simulink model "cuurent_controlled_circuit"  (R2022a)
settings: Solver=VariableStepAuto  StartTime=0.0  StopTime=25.0  RelTol=1e-3
undefined symbols (not defined in the file or in its folder): DiscIntNeverNeededParam
libraries: fl_lib x82, nesl_utility x65, eeRmsMeasurement x34, eePowerMeasurement x17, ee_lib x16
(part 3 of 3)

== system cuurent_controlled_circuit/Subsystem5 ==
  Display3 : Display
  Display4 : Display
  Display5 : Display
  PS-Simulink Converter2 : nesl_utility/PS-Simulink Converter  PhysicalDomain=network_engine_domain  SubClassName=ps_output  LeftPortType=input  RightPortType=output  PseudoPeriodic=off  Frequencies=[]  VectorFormat=inherit  Unit=inherit  AffineConversion=off
      settings: SourceProductBaseCode=SS,PW,VE
  PS-Simulink Converter3 : nesl_utility/PS-Simulink Converter  PhysicalDomain=network_engine_domain  SubClassName=ps_output  LeftPortType=input  RightPortType=output  PseudoPeriodic=off  Frequencies=[]  VectorFormat=inherit  Unit=inherit  AffineConversion=off
      settings: SourceProductBaseCode=SS,PW,VE
  Power Measurement2 : eePowerMeasurement/Power Measurement  LabelModeActiveChoice=Continuous  F=50  K=[0 1 2 3]  Ts=0
      settings: SourceProductBaseCode=PS
  RMS Measurement2 : eeRmsMeasurement/RMS Measurement  LabelModeActiveChoice=Total  F=50  SpecifyHarmonics=off  K=[0 1 2]  Ts=0
      settings: SourceProductBaseCode=PS
  RMS Measurement3 : eeRmsMeasurement/RMS Measurement  LabelModeActiveChoice=Total  F=50  SpecifyHarmonics=off  K=[0 1 2]  Ts=0
      settings: SourceProductBaseCode=PS
  Scope{6..10} (5 alike) : Scope
  input : PMIOPort  Side=Left
  input1 : PMIOPort  Port=2  Side=Left
  Q : Outport
  wires:
  Power Measurement2/2 -> Q/1
  PS-Simulink Converter3/1 -> RMS Measurement3/1, Scope8/1
  Power Measurement2/1 -> Display5/1, Scope10/1
  RMS Measurement2/1 -> Scope7/1, Display3/1, Power Measurement2/1
  PS-Simulink Converter2/1 -> RMS Measurement2/1, Scope6/1
  RMS Measurement3/1 -> Power Measurement2/2, Scope9/1, Display4/1
  connections:
  PS-Simulink Converter3/LConn1 -- input1/RConn1
  PS-Simulink Converter2/LConn1 -- input/RConn1

== system cuurent_controlled_circuit/Subsystem6 ==
  Display3 : Display
  Display4 : Display
  Display5 : Display
  PS-Simulink Converter2 : nesl_utility/PS-Simulink Converter  PhysicalDomain=network_engine_domain  SubClassName=ps_output  LeftPortType=input  RightPortType=output  PseudoPeriodic=off  Frequencies=[]  VectorFormat=inherit  Unit=inherit  AffineConversion=off
      settings: SourceProductBaseCode=SS,PW,VE
  PS-Simulink Converter3 : nesl_utility/PS-Simulink Converter  PhysicalDomain=network_engine_domain  SubClassName=ps_output  LeftPortType=input  RightPortType=output  PseudoPeriodic=off  Frequencies=[]  VectorFormat=inherit  Unit=inherit  AffineConversion=off
      settings: SourceProductBaseCode=SS,PW,VE
  Power Measurement2 : eePowerMeasurement/Power Measurement  LabelModeActiveChoice=Continuous  F=50  K=[0 1 2 3]  Ts=0
      settings: SourceProductBaseCode=PS
  RMS Measurement2 : eeRmsMeasurement/RMS Measurement  LabelModeActiveChoice=Total  F=50  SpecifyHarmonics=off  K=[0 1 2]  Ts=0
      settings: SourceProductBaseCode=PS
  RMS Measurement3 : eeRmsMeasurement/RMS Measurement  LabelModeActiveChoice=Total  F=50  SpecifyHarmonics=off  K=[0 1 2]  Ts=0
      settings: SourceProductBaseCode=PS
  Scope{6..10} (5 alike) : Scope
  input : PMIOPort  Side=Left
  input1 : PMIOPort  Port=2  Side=Left
  Q : Outport
  wires:
  Power Measurement2/2 -> Q/1
  PS-Simulink Converter3/1 -> RMS Measurement3/1, Scope8/1
  Power Measurement2/1 -> Display5/1, Scope10/1
  RMS Measurement2/1 -> Scope7/1, Display3/1, Power Measurement2/1
  PS-Simulink Converter2/1 -> RMS Measurement2/1, Scope6/1
  RMS Measurement3/1 -> Power Measurement2/2, Scope9/1, Display4/1
  connections:
  PS-Simulink Converter3/LConn1 -- input1/RConn1
  PS-Simulink Converter2/LConn1 -- input/RConn1

== system cuurent_controlled_circuit/Subsystem7 ==
  Display3 : Display
  Display4 : Display
  Display5 : Display
  PS-Simulink Converter2 : nesl_utility/PS-Simulink Converter  PhysicalDomain=network_engine_domain  SubClassName=ps_output  LeftPortType=input  RightPortType=output  PseudoPeriodic=off  Frequencies=[]  VectorFormat=inherit  Unit=inherit  AffineConversion=off
      settings: SourceProductBaseCode=SS,PW,VE
  PS-Simulink Converter3 : nesl_utility/PS-Simulink Converter  PhysicalDomain=network_engine_domain  SubClassName=ps_output  LeftPortType=input  RightPortType=output  PseudoPeriodic=off  Frequencies=[]  VectorFormat=inherit  Unit=inherit  AffineConversion=off
      settings: SourceProductBaseCode=SS,PW,VE
  Power Measurement2 : eePowerMeasurement/Power Measurement  LabelModeActiveChoice=Continuous  F=50  K=[0 1 2 3]  Ts=0
      settings: SourceProductBaseCode=PS
  RMS Measurement2 : eeRmsMeasurement/RMS Measurement  LabelModeActiveChoice=Total  F=50  SpecifyHarmonics=off  K=[0 1 2]  Ts=0
      settings: SourceProductBaseCode=PS
  RMS Measurement3 : eeRmsMeasurement/RMS Measurement  LabelModeActiveChoice=Total  F=50  SpecifyHarmonics=off  K=[0 1 2]  Ts=0
      settings: SourceProductBaseCode=PS
  Scope{6..10} (5 alike) : Scope
  input : PMIOPort  Side=Left
  input1 : PMIOPort  Port=2  Side=Left
  Q : Outport
  wires:
  Power Measurement2/2 -> Q/1
  PS-Simulink Converter3/1 -> RMS Measurement3/1, Scope8/1
  Power Measurement2/1 -> Display5/1, Scope10/1
  RMS Measurement2/1 -> Scope7/1, Display3/1, Power Measurement2/1
  PS-Simulink Converter2/1 -> RMS Measurement2/1, Scope6/1
  RMS Measurement3/1 -> Power Measurement2/2, Scope9/1, Display4/1
  connections:
  PS-Simulink Converter3/LConn1 -- input1/RConn1
  PS-Simulink Converter2/LConn1 -- input/RConn1

== system cuurent_controlled_circuit/Subsystem8 ==
  Display3 : Display
  Display4 : Display
  Display5 : Display
  PS-Simulink Converter2 : nesl_utility/PS-Simulink Converter  PhysicalDomain=network_engine_domain  SubClassName=ps_output  LeftPortType=input  RightPortType=output  PseudoPeriodic=off  Frequencies=[]  VectorFormat=inherit  Unit=inherit  AffineConversion=off
      settings: SourceProductBaseCode=SS,PW,VE
  PS-Simulink Converter3 : nesl_utility/PS-Simulink Converter  PhysicalDomain=network_engine_domain  SubClassName=ps_output  LeftPortType=input  RightPortType=output  PseudoPeriodic=off  Frequencies=[]  VectorFormat=inherit  Unit=inherit  AffineConversion=off
      settings: SourceProductBaseCode=SS,PW,VE
  Power Measurement2 : eePowerMeasurement/Power Measurement  LabelModeActiveChoice=Continuous  F=50  K=[0 1 2 3]  Ts=0
      settings: SourceProductBaseCode=PS
  RMS Measurement2 : eeRmsMeasurement/RMS Measurement  LabelModeActiveChoice=Total  F=50  SpecifyHarmonics=off  K=[0 1 2]  Ts=0
      settings: SourceProductBaseCode=PS
  RMS Measurement3 : eeRmsMeasurement/RMS Measurement  LabelModeActiveChoice=Total  F=50  SpecifyHarmonics=off  K=[0 1 2]  Ts=0
      settings: SourceProductBaseCode=PS
  Scope{6..10} (5 alike) : Scope
  input : PMIOPort  Side=Left
  input1 : PMIOPort  Port=2  Side=Left
  Q : Outport
  wires:
  Power Measurement2/2 -> Q/1
  PS-Simulink Converter3/1 -> RMS Measurement3/1, Scope8/1
  Power Measurement2/1 -> Display5/1, Scope10/1
  RMS Measurement2/1 -> Scope7/1, Display3/1, Power Measurement2/1
  PS-Simulink Converter2/1 -> RMS Measurement2/1, Scope6/1
  RMS Measurement3/1 -> Power Measurement2/2, Scope9/1, Display4/1
  connections:
  PS-Simulink Converter3/LConn1 -- input1/RConn1
  PS-Simulink Converter2/LConn1 -- input/RConn1

== system cuurent_controlled_circuit/Subsystem9 ==
  Display3 : Display
  Display4 : Display
  Display5 : Display
  PS-Simulink Converter2 : nesl_utility/PS-Simulink Converter  PhysicalDomain=network_engine_domain  SubClassName=ps_output  LeftPortType=input  RightPortType=output  PseudoPeriodic=off  Frequencies=[]  VectorFormat=inherit  Unit=inherit  AffineConversion=off
      settings: SourceProductBaseCode=SS,PW,VE
  PS-Simulink Converter3 : nesl_utility/PS-Simulink Converter  PhysicalDomain=network_engine_domain  SubClassName=ps_output  LeftPortType=input  RightPortType=output  PseudoPeriodic=off  Frequencies=[]  VectorFormat=inherit  Unit=inherit  AffineConversion=off
      settings: SourceProductBaseCode=SS,PW,VE
  Power Measurement2 : eePowerMeasurement/Power Measurement  LabelModeActiveChoice=Continuous  F=50  K=[0 1 2 3]  Ts=0
      settings: SourceProductBaseCode=PS
  RMS Measurement2 : eeRmsMeasurement/RMS Measurement  LabelModeActiveChoice=Total  F=50  SpecifyHarmonics=off  K=[0 1 2]  Ts=0
      settings: SourceProductBaseCode=PS
  RMS Measurement3 : eeRmsMeasurement/RMS Measurement  LabelModeActiveChoice=Total  F=50  SpecifyHarmonics=off  K=[0 1 2]  Ts=0
      settings: SourceProductBaseCode=PS
  Scope{6..10} (5 alike) : Scope
  input : PMIOPort  Side=Left
  input1 : PMIOPort  Port=2  Side=Left
  Q : Outport
  wires:
  Power Measurement2/2 -> Q/1
  PS-Simulink Converter3/1 -> RMS Measurement3/1, Scope8/1
  Power Measurement2/1 -> Display5/1, Scope10/1
  RMS Measurement2/1 -> Scope7/1, Display3/1, Power Measurement2/1
  PS-Simulink Converter2/1 -> RMS Measurement2/1, Scope6/1
  RMS Measurement3/1 -> Power Measurement2/2, Scope9/1, Display4/1
  connections:
  PS-Simulink Converter3/LConn1 -- input1/RConn1
  PS-Simulink Converter2/LConn1 -- input/RConn1

== matlab function cuurent_controlled_circuit/Subsystem27/MATLAB Function4 ==
  data: pvandwind input; charge output; load input; discharge output; batterycharge input
function [charge,discharge] = fcn(pvandwind,load,batterycharge)

if (pvandwind-load)>0 && (batterycharge<95)
    charge=pvandwind-load;
    discharge=0;

elseif (batterycharge>15) && (pvandwind-load)<=0
    charge=0;
    discharge=load-pvandwind;
else
     charge=0;
    discharge=0;
end

== matlab function cuurent_controlled_circuit/Subsystem20/MATLAB Function4 ==
  data: pvandwind input; charge output; load input; discharge output; batterycharge input
function [charge,discharge] = fcn(pvandwind,load,batterycharge)

if (pvandwind-load)>0 && (batterycharge<95)
    charge=pvandwind-load;
    discharge=0;

elseif (batterycharge>15) && (pvandwind-load)<=0
    charge=0;
    discharge=load-pvandwind;
else
     charge=0;
    discharge=0;
end

== matlab function cuurent_controlled_circuit/Subsystem28/MATLAB Function4 ==
  data: pvandwind input; charge output; load input; discharge output; batterycharge input
function [charge,discharge] = fcn(pvandwind,load,batterycharge)

if (pvandwind-load)>0 && (batterycharge<95)
    charge=pvandwind-load;
    discharge=0;

elseif (batterycharge>15) && (pvandwind-load)<=0
    charge=0;
    discharge=load-pvandwind;
else
     charge=0;
    discharge=0;
end

== matlab function cuurent_controlled_circuit/Subsystem29/MATLAB Function4 ==
  data: pvandwind input; charge output; load input; discharge output; batterycharge input
function [charge,discharge] = fcn(pvandwind,load,batterycharge)

if (pvandwind-load)>0 && (batterycharge<95)
    charge=pvandwind-load;
    discharge=0;

elseif (batterycharge>15) && (pvandwind-load)<=0
    charge=0;
    discharge=load-pvandwind;
else
     charge=0;
    discharge=0;
end

== matlab function cuurent_controlled_circuit/Subsystem30/MATLAB Function4 ==
  data: pvandwind input; charge output; load input; discharge output; batterycharge input
function [charge,discharge] = fcn(pvandwind,load,batterycharge)

if (pvandwind-load)>0 && (batterycharge<95)
    charge=pvandwind-load;
    discharge=0;

elseif (batterycharge>15) && (pvandwind-load)<=0
    charge=0;
    discharge=load-pvandwind;
else
     charge=0;
    discharge=0;
end

== matlab function cuurent_controlled_circuit/Subsystem31/MATLAB Function4 ==
  data: pvandwind input; charge output; load input; discharge output; batterycharge input
function [charge,discharge] = fcn(pvandwind,load,batterycharge)

if (pvandwind-load)>0 && (batterycharge<95)
    charge=pvandwind-load;
    discharge=0;

elseif (batterycharge>15) && (pvandwind-load)<=0
    charge=0;
    discharge=load-pvandwind;
else
     charge=0;
    discharge=0;
end

== matlab function cuurent_controlled_circuit/Subsystem32/MATLAB Function4 ==
  data: pvandwind input; charge output; load input; discharge output; batterycharge input
function [charge,discharge] = fcn(pvandwind,load,batterycharge)

if (pvandwind-load)>0 && (batterycharge<95)
    charge=pvandwind-load;
    discharge=0;

elseif (batterycharge>15) && (pvandwind-load)<=0
    charge=0;
    discharge=load-pvandwind;
else
     charge=0;
    discharge=0;
end

== matlab function cuurent_controlled_circuit/Subsystem16/MATLAB Function4 ==
  data: pvandwind input; charge output; load input; discharge output; batterycharge input
function [charge,discharge] = fcn(pvandwind,load,batterycharge)

if (pvandwind-load)>0 && (batterycharge<95)
    charge=pvandwind-load;
    discharge=0;

elseif (batterycharge>15) && (pvandwind-load)<=0
    charge=0;
    discharge=load-pvandwind;
else
     charge=0;
    discharge=0;
end

== matlab function cuurent_controlled_circuit/Subsystem21/MATLAB Function4 ==
  data: pvandwind input; charge output; load input; discharge output; batterycharge input
function [charge,discharge] = fcn(pvandwind,load,batterycharge)

if (pvandwind-load)>0 && (batterycharge<95)
    charge=pvandwind-load;
    discharge=0;

elseif (batterycharge>15) && (pvandwind-load)<=0
    charge=0;
    discharge=load-pvandwind;
else
     charge=0;
    discharge=0;
end

== matlab function cuurent_controlled_circuit/Subsystem22/MATLAB Function4 ==
  data: pvandwind input; charge output; load input; discharge output; batterycharge input
function [charge,discharge] = fcn(pvandwind,load,batterycharge)

if (pvandwind-load)>0 && (batterycharge<95)
    charge=pvandwind-load;
    discharge=0;

elseif (batterycharge>15) && (pvandwind-load)<=0
    charge=0;
    discharge=load-pvandwind;
else
     charge=0;
    discharge=0;
end

== matlab function cuurent_controlled_circuit/Subsystem19/Battery Management System ==
  data: pvandwind input; charge output; load input; discharge output; batterycharge input
function [charge,discharge] = fcn(pvandwind,load,batterycharge)

if (pvandwind-load)>0 && (batterycharge<95)
    charge=pvandwind-load;
    discharge=0;

elseif (batterycharge>15) && (pvandwind-load)<=0
    charge=0;
    discharge=load-pvandwind;
else
     charge=0;
    discharge=0;
end

== matlab function cuurent_controlled_circuit/Subsystem23/MATLAB Function4 ==
  data: pvandwind input; charge output; load input; discharge output; batterycharge input
function [charge,discharge] = fcn(pvandwind,load,batterycharge)

if (pvandwind-load)>0 && (batterycharge<95)
    charge=pvandwind-load;
    discharge=0;

elseif (batterycharge>15) && (pvandwind-load)<=0
    charge=0;
    discharge=load-pvandwind;
else
     charge=0;
    discharge=0;
end

== matlab function cuurent_controlled_circuit/Subsystem24/MATLAB Function4 ==
  data: pvandwind input; charge output; load input; discharge output; batterycharge input
function [charge,discharge] = fcn(pvandwind,load,batterycharge)

if (pvandwind-load)>0 && (batterycharge<95)
    charge=pvandwind-load;
    discharge=0;

elseif (batterycharge>15) && (pvandwind-load)<=0
    charge=0;
    discharge=load-pvandwind;
else
     charge=0;
    discharge=0;
end

== matlab function cuurent_controlled_circuit/Subsystem25/MATLAB Function4 ==
  data: pvandwind input; charge output; load input; discharge output; batterycharge input
function [charge,discharge] = fcn(pvandwind,load,batterycharge)

if (pvandwind-load)>0 && (batterycharge<95)
    charge=pvandwind-load;
    discharge=0;

elseif (batterycharge>15) && (pvandwind-load)<=0
    charge=0;
    discharge=load-pvandwind;
else
     charge=0;
    discharge=0;
end

== matlab function cuurent_controlled_circuit/Subsystem26/MATLAB Function4 ==
  data: pvandwind input; charge output; load input; discharge output; batterycharge input
function [charge,discharge] = fcn(pvandwind,load,batterycharge)

if (pvandwind-load)>0 && (batterycharge<95)
    charge=pvandwind-load;
    discharge=0;

elseif (batterycharge>15) && (pvandwind-load)<=0
    charge=0;
    discharge=load-pvandwind;
else
     charge=0;
    discharge=0;
end
